simulink model "diff_eq2"  (R2020b)
settings: Solver=VariableStepAuto  StartTime=0.0  StopTime=10.0  RelTol=1e-3
values from neighbouring files (symbols this model uses):
  y = 2    [diff_code2.m]
settings Model: Creator=amnessa  LastModifiedBy=amnessa

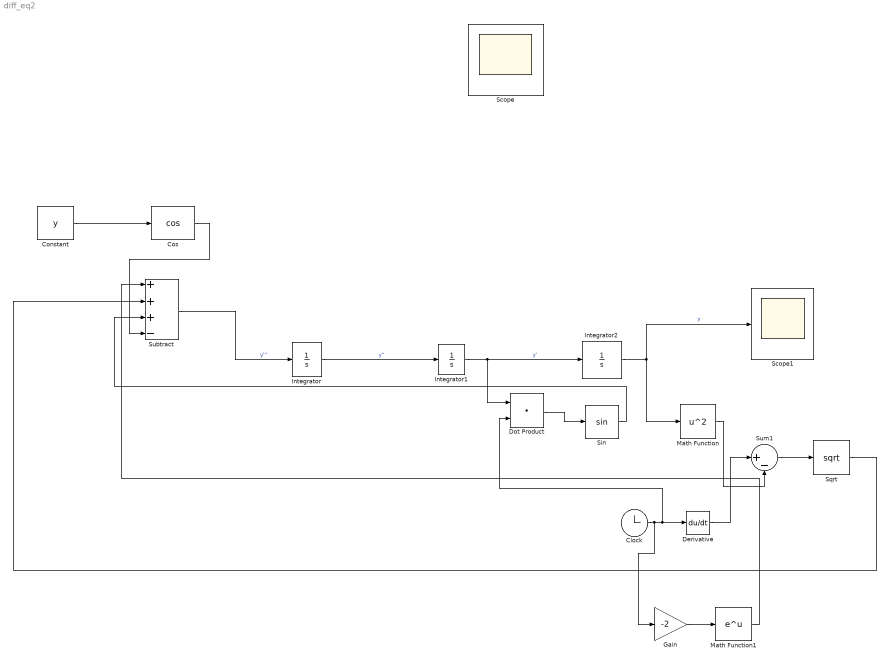
== system diff_eq2 ==
  Clock : Clock
  Constant : Constant  Value=y
  Cos : Trigonometry  Operator=cos
  Derivative : Derivative
  Dot Product : DotProduct  InputSameDT=on  OutDataTypeStr=Inherit: Inherit via internal rule
  Gain : Gain  Gain=-2
  Integrator : Integrator
  Integrator1 : Integrator
  Integrator2 : Integrator
  Math Function : Math  Operator=square  SaturateOnIntegerOverflow=on
  Math Function1 : Math  SaturateOnIntegerOverflow=on
  Scope : Scope
  Scope1 : Scope
  Sin : Trigonometry
  Sqrt : Sqrt  SaturateOnIntegerOverflow=on
  Subtract : Sum  Inputs=+++-
  Sum1 : Sum  Inputs=|+-
  wires:
  Integrator/1 -> Integrator1/1  "y''"
  Integrator1/1 -> Dot Product/1, Integrator2/1  "y'"
  Integrator2/1 -> Math Function/1, Scope1/1  "y"
  Subtract/1 -> Integrator/1  "y'''"
  Sin/1 -> Subtract/3
  Constant/1 -> Cos/1
  Cos/1 -> Subtract/4
  Clock/1 -> Gain/1, Dot Product/2, Derivative/1
  Derivative/1 -> Sum1/1
  Math Function/1 -> Sum1/2
  Dot Product/1 -> Sin/1
  Sum1/1 -> Sqrt/1
  Sqrt/1 -> Subtract/2
  Gain/1 -> Math Function1/1
  Math Function1/1 -> Subtract/1
